simulink model "QPSK_Transmit_v5_w_FIFO_w_errors"  (R2012b)
settings: Solver=FixedStepDiscrete  StartTime=0.0  StopTime=1500  FixedStep=1  RelTol=1e-3
libraries: simulink x14, dspbuff3 x1, commutil2 x1
settings Model: Creator=Carl  LastModifiedBy=Carl
settings DataIOCC: SignalLogging=off
settings OptimizationCC: BlockReduction=off  ConditionallyExecuteInputs=off  InlineParams=on
settings DebuggingCC: AlgebraicLoopMsg=error
settings HardwareCC: ProdHWDeviceType=ASIC/FPGA->ASIC/FPGA  ProdEqTarget=off

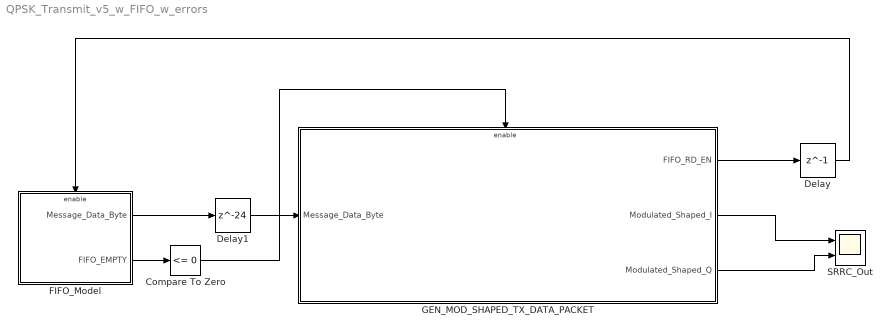
== system QPSK_Transmit_v5_w_FIFO_w_errors ==
  Compare To Zero : simulink/Logic and Bit Operations/Compare To Zero  relop=<=  OutDataTypeStr=boolean
  Delay : Delay  DelayLength=1  InitialCondition=0
  Delay1 : Delay  DelayLength=24  InitialCondition=0
  FIFO_Model : Subsystem
  GEN_MOD_SHAPED_TX_DATA_PACKET : Subsystem
  SRRC_Out : Scope  NumInputPorts=2
      settings: YMin=-5~-5  YMax=5~5  SaveName=ScopeData7
  wires:
  GEN_MOD_SHAPED_TX_DATA_PACKET/2(Modulated_Shaped_I) -> SRRC_Out/1
  GEN_MOD_SHAPED_TX_DATA_PACKET/3(Modulated_Shaped_Q) -> SRRC_Out/2
  GEN_MOD_SHAPED_TX_DATA_PACKET/1(FIFO_RD_EN) -> Delay/1
  Delay/1 -> FIFO_Model/Enable
  FIFO_Model/2(FIFO_EMPTY) -> Compare To Zero/1
  Compare To Zero/1 -> GEN_MOD_SHAPED_TX_DATA_PACKET/Enable
  FIFO_Model/1(Message_Data_Byte) -> Delay1/1
  Delay1/1 -> GEN_MOD_SHAPED_TX_DATA_PACKET/1(Message_Data_Byte)

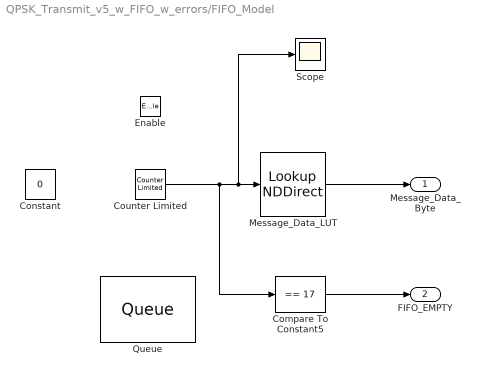
== system QPSK_Transmit_v5_w_FIFO_w_errors/FIFO_Model ==
  Enable : EnablePort
  Compare To Constant5 : simulink/Logic and Bit Operations/Compare To Constant  relop===  const=17  OutDataTypeStr=boolean  ZeroCross=off
  Constant : Constant  Value=0
  Counter Limited : simulink/Sources/Counter Limited  uplimit=17  tsamp=-1
  Message_Data_LUT : LookupNDDirect  NumberOfTableDimensions=1  Table="[12        0        0        1        104        101        108        108        111        32        119        111        114        108        100        33        198        228]"  DiagnosticForOutOfRangeInput=Error  TableDataTypeStr=uint8
  Queue : dspbuff3/Queue  depth=8  trigger=Rising edge  overflow=Dynamic reallocation  pes=Warning  eso=off  fso=off  nso=off  clr=off  clrOutport=off  adf=on
  Scope : Scope
  Message_Data_Byte : Outport
  FIFO_EMPTY : Outport  Port=2
  wires:
  Message_Data_LUT/1 -> Message_Data_Byte/1
  Counter Limited/1 -> Compare To Constant5/1, Scope/1, Message_Data_LUT/1
  Compare To Constant5/1 -> FIFO_EMPTY/1

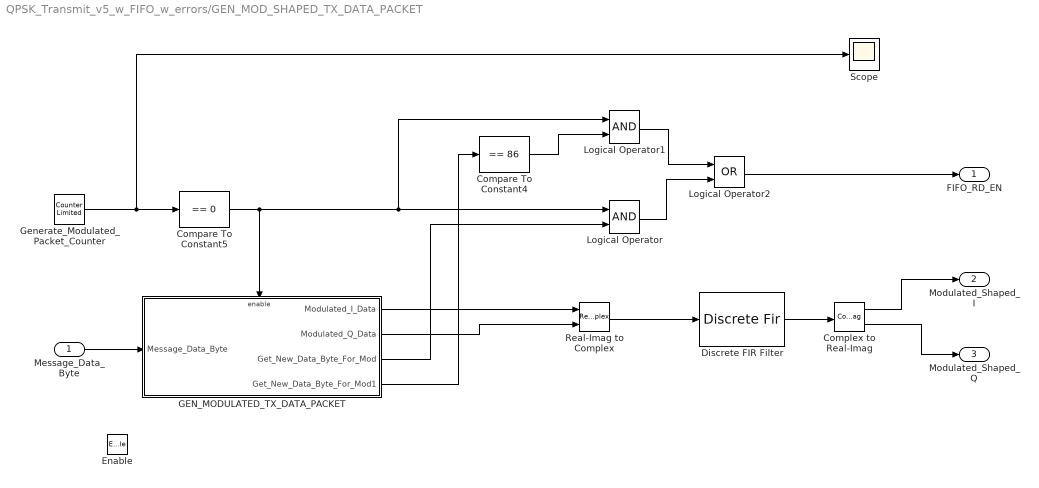
== system QPSK_Transmit_v5_w_FIFO_w_errors/GEN_MOD_SHAPED_TX_DATA_PACKET ==
  Message_Data_Byte : Inport
  Enable : EnablePort
  Compare To Constant4 : simulink/Logic and Bit Operations/Compare To Constant  relop===  const=86  OutDataTypeStr=boolean  ZeroCross=off
  Compare To Constant5 : simulink/Logic and Bit Operations/Compare To Constant  relop===  const=0  OutDataTypeStr=boolean  ZeroCross=off
  Complex to Real-Imag : ComplexToRealImag
  Discrete FIR Filter : DiscreteFir  Coefficients=|
      | [
      | 0.006690562067
      | -0.005768593810
      | -0.011827354519
      | 0.020586915021
      | 0.016726405168
      | -0.053692342207
      | -0.020253031546
      | 0.196043589067
      | 0.336822413190
      | 0.196043589067
      | -0.020253031546
      | -0.053692342207
      | 0.016726405168
      | 0.020586915021
      | -0.011827354519
      | -0.005768593810
      | 0.006690562067
      | ]
  GEN_MODULATED_TX_DATA_PACKET : Subsystem
  Generate_Modulated_Packet_Counter : simulink/Sources/Counter Limited  uplimit=7  tsamp=-1
  Logical Operator : Logic  AllPortsSameDT=off  OutDataTypeStr=boolean
  Logical Operator1 : Logic  AllPortsSameDT=off  OutDataTypeStr=boolean
  Logical Operator2 : Logic  Operator=OR  AllPortsSameDT=off  OutDataTypeStr=boolean
  Real-Imag to Complex : RealImagToComplex
  Scope : Scope
      settings: SaveName=ScopeData10
  FIFO_RD_EN : Outport
  Modulated_Shaped_I : Outport  Port=2
  Modulated_Shaped_Q : Outport  Port=3
  wires:
  Real-Imag to Complex/1 -> Discrete FIR Filter/1
  Discrete FIR Filter/1 -> Complex to Real-Imag/1
  Complex to Real-Imag/1 -> Modulated_Shaped_I/1
  Complex to Real-Imag/2 -> Modulated_Shaped_Q/1
  GEN_MODULATED_TX_DATA_PACKET/1(Modulated_I_Data) -> Real-Imag to Complex/1
  GEN_MODULATED_TX_DATA_PACKET/2(Modulated_Q_Data) -> Real-Imag to Complex/2
  Generate_Modulated_Packet_Counter/1 -> Scope/1, Compare To Constant5/1
  Message_Data_Byte/1 -> GEN_MODULATED_TX_DATA_PACKET/1(Message_Data_Byte)
  GEN_MODULATED_TX_DATA_PACKET/3(Get_New_Data_Byte_For_Mod) -> Logical Operator/2
  Compare To Constant5/1 -> GEN_MODULATED_TX_DATA_PACKET/Enable, Logical Operator1/1, Logical Operator/1
  Compare To Constant4/1 -> Logical Operator1/2
  GEN_MODULATED_TX_DATA_PACKET/4(Get_New_Data_Byte_For_Mod1) -> Compare To Constant4/1
  Logical Operator/1 -> Logical Operator2/2
  Logical Operator1/1 -> Logical Operator2/1
  Logical Operator2/1 -> FIFO_RD_EN/1

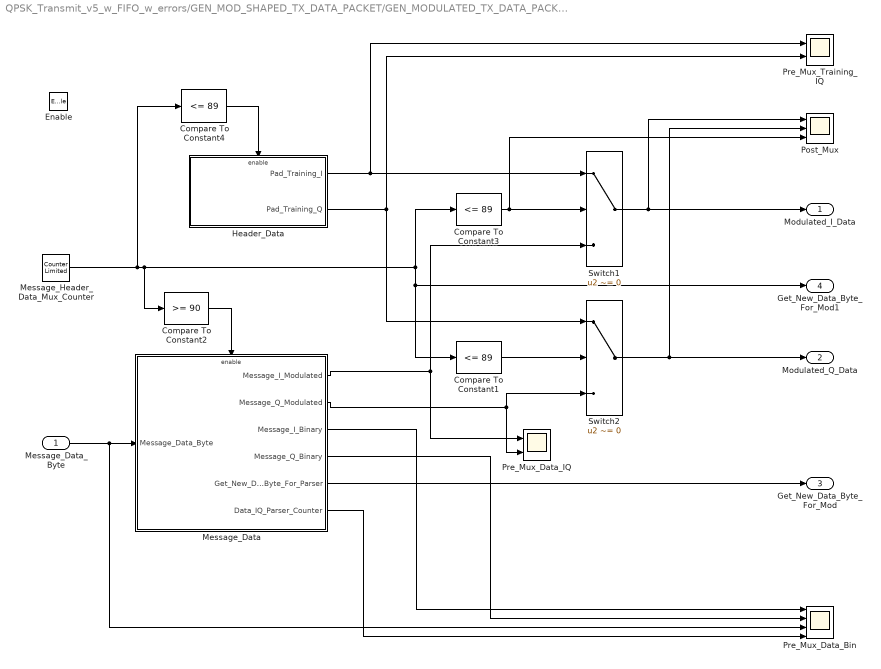
== system QPSK_Transmit_v5_w_FIFO_w_errors/GEN_MOD_SHAPED_TX_DATA_PACKET/GEN_MODULATED_TX_DATA_PACKET ==
  Message_Data_Byte : Inport
  Enable : EnablePort
  Compare To Constant1 : simulink/Logic and Bit Operations/Compare To Constant  relop=<=  const=89  OutDataTypeStr=boolean  ZeroCross=off
  Compare To Constant2 : simulink/Logic and Bit Operations/Compare To Constant  relop=>=  const=90  OutDataTypeStr=boolean  ZeroCross=off
  Compare To Constant3 : simulink/Logic and Bit Operations/Compare To Constant  relop=<=  const=89  OutDataTypeStr=boolean  ZeroCross=off
  Compare To Constant4 : simulink/Logic and Bit Operations/Compare To Constant  relop=<=  const=89  OutDataTypeStr=boolean  ZeroCross=off
  Header_Data : Subsystem
  Message_Data : Subsystem
  Message_Header_Data_Mux_Counter : simulink/Sources/Counter Limited  uplimit=1023  tsamp=-1
  Post_Mux : Scope  NumInputPorts=3
      settings: YMin=-5~-5~-5  YMax=5~5~5  SaveName=ScopeData2
  Pre_Mux_Data_Bin : Scope  NumInputPorts=4
      settings: TimeRange=1500  YMin=-0.2~-0.2~-10~-5  YMax=1.2~1.2~265~5  SaveName=ScopeData6
  Pre_Mux_Data_IQ : Scope  NumInputPorts=2
      settings: YMin=-5~-5  YMax=5~5  SaveName=ScopeData5
  Pre_Mux_Training_IQ : Scope  NumInputPorts=2
      settings: YMin=-5~-5  YMax=5~5  SaveName=ScopeData4
  Switch1 : Switch  Criteria=u2 ~= 0  OutDataTypeStr=int8
  Switch2 : Switch  Criteria=u2 ~= 0  OutDataTypeStr=int8
  Modulated_I_Data : Outport
  Modulated_Q_Data : Outport  Port=2
  Get_New_Data_Byte_For_Mod : Outport  Port=3
  Get_New_Data_Byte_For_Mod1 : Outport  Port=4
  wires:
  Message_Header_Data_Mux_Counter/1 -> Compare To Constant4/1, Compare To Constant3/1, Get_New_Data_Byte_For_Mod1/1, Compare To Constant1/1, Compare To Constant2/1
  Switch1/1 -> Modulated_I_Data/1, Post_Mux/1
  Header_Data/1(Pad_Training_I) -> Switch1/1, Pre_Mux_Training_IQ/1
  Compare To Constant1/1 -> Switch2/2
  Switch2/1 -> Post_Mux/2, Modulated_Q_Data/1
  Header_Data/2(Pad_Training_Q) -> Switch2/1, Pre_Mux_Training_IQ/2
  Message_Data/2(Message_Q_Modulated) -> Pre_Mux_Data_IQ/2, Switch2/3
  Message_Data/1(Message_I_Modulated) -> Pre_Mux_Data_IQ/1, Switch1/3
  Message_Data/3(Message_I_Binary) -> Pre_Mux_Data_Bin/1
  Message_Data/4(Message_Q_Binary) -> Pre_Mux_Data_Bin/2
  Compare To Constant2/1 -> Message_Data/Enable
  Compare To Constant4/1 -> Header_Data/Enable
  Message_Data_Byte/1 -> Pre_Mux_Data_Bin/3, Message_Data/1(Message_Data_Byte)
  Compare To Constant3/1 -> Post_Mux/3, Switch1/2
  Message_Data/5(Get_New_Data_Byte_For_Parser) -> Get_New_Data_Byte_For_Mod/1
  Message_Data/6(Data_IQ_Parser_Counter) -> Pre_Mux_Data_Bin/4

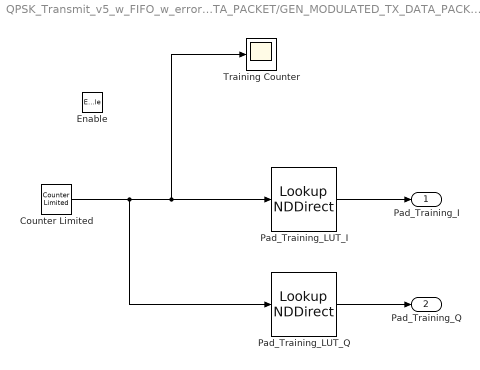
== system QPSK_Transmit_v5_w_FIFO_w_errors/GEN_MOD_SHAPED_TX_DATA_PACKET/GEN_MODULATED_TX_DATA_PACKET/Header_Data ==
  Enable : EnablePort
  Counter Limited : simulink/Sources/Counter Limited  uplimit=89  tsamp=-1
  Pad_Training_LUT_I : LookupNDDirect  NumberOfTableDimensions=1  Table=[1,-1,1,-1,1,-1,1,-1,1,-1,1,-1,1,-1,1,-1,1,-1,1,-1,1,-1,1,-1,1,1,1,-1,-1,1,1,-1,-1,1,-1,-1,-1,-1,1,-1,1,1,-1,-1,1,1,1,-1,1,1,1,-1,1,-1,1,1,1,-1,1,1,1,1,-1,1,1,-1,-1,-1,-1,1,1,1,-1,-1,-1,1,1,1,1,-1,1,1,1,1,1,-1,-1,-1,1,1]  DiagnosticForOutOfRangeInput=Error  TableDataTypeStr=int8
  Pad_Training_LUT_Q : LookupNDDirect  NumberOfTableDimensions=1  Table=[1,-1,1,-1,1,-1,1,-1,1,-1,1,-1,1,-1,1,-1,1,-1,1,-1,1,-1,1,-1,1,1,-1,1,1,1,-1,-1,-1,-1,1,1,-1,1,1,-1,-1,-1,1,-1,-1,1,1,1,-1,-1,1,1,1,-1,-1,-1,-1,-1,-1,1,1,-1,1,-1,1,1,-1,-1,1,-1,-1,1,1,-1,-1,-1,-1,-1,1,1,1,1,-1,-1,-1,-1,1,-1,1,-1]  DiagnosticForOutOfRangeInput=Error  TableDataTypeStr=int8
  Training Counter : Scope
      settings: SaveName=ScopeData3
  Pad_Training_I : Outport
  Pad_Training_Q : Outport  Port=2
  wires:
  Pad_Training_LUT_I/1 -> Pad_Training_I/1
  Counter Limited/1 -> Training Counter/1, Pad_Training_LUT_I/1, Pad_Training_LUT_Q/1
  Pad_Training_LUT_Q/1 -> Pad_Training_Q/1

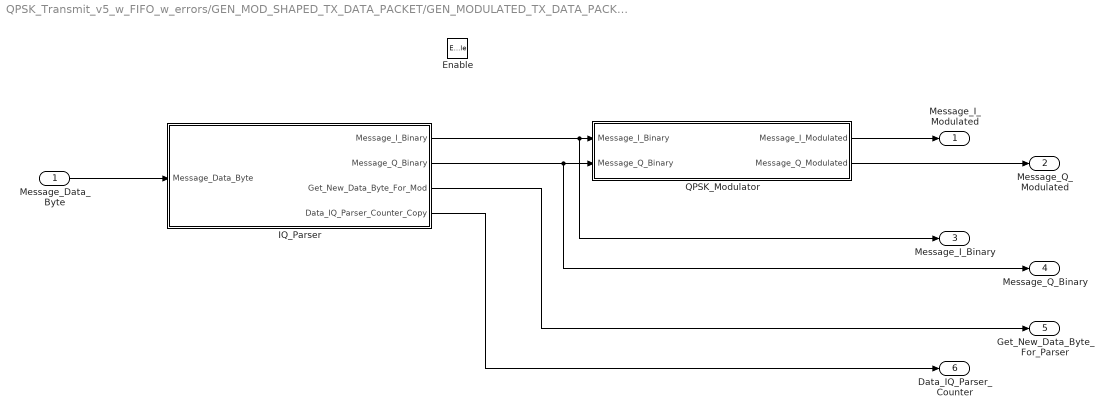
== system QPSK_Transmit_v5_w_FIFO_w_errors/GEN_MOD_SHAPED_TX_DATA_PACKET/GEN_MODULATED_TX_DATA_PACKET/Message_Data ==
  Message_Data_Byte : Inport
  Enable : EnablePort
  IQ_Parser : Subsystem
  QPSK_Modulator : Subsystem
  Message_I_Modulated : Outport
  Message_Q_Modulated : Outport  Port=2
  Message_I_Binary : Outport  Port=3
  Message_Q_Binary : Outport  Port=4
  Get_New_Data_Byte_For_Parser : Outport  Port=5
  Data_IQ_Parser_Counter : Outport  Port=6
  wires:
  IQ_Parser/1(Message_I_Binary) -> Message_I_Binary/1, QPSK_Modulator/1(Message_I_Binary)
  IQ_Parser/2(Message_Q_Binary) -> Message_Q_Binary/1, QPSK_Modulator/2(Message_Q_Binary)
  QPSK_Modulator/1(Message_I_Modulated) -> Message_I_Modulated/1
  QPSK_Modulator/2(Message_Q_Modulated) -> Message_Q_Modulated/1
  Message_Data_Byte/1 -> IQ_Parser/1(Message_Data_Byte)
  IQ_Parser/3(Get_New_Data_Byte_For_Mod) -> Get_New_Data_Byte_For_Parser/1
  IQ_Parser/4(Data_IQ_Parser_Counter_Copy) -> Data_IQ_Parser_Counter/1

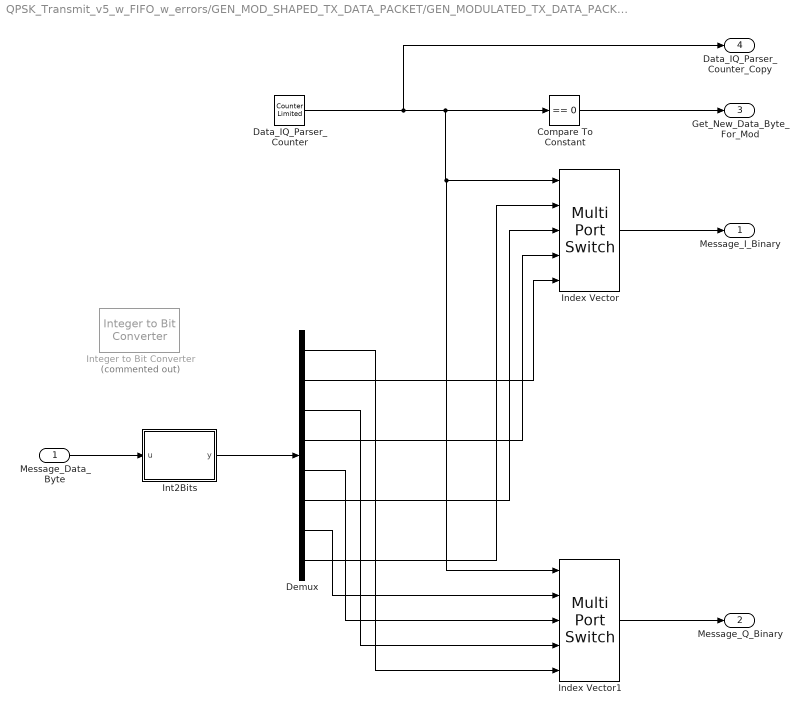
== system QPSK_Transmit_v5_w_FIFO_w_errors/GEN_MOD_SHAPED_TX_DATA_PACKET/GEN_MODULATED_TX_DATA_PACKET/Message_Data/IQ_Parser ==
  Message_Data_Byte : Inport
  Compare To Constant : simulink/Logic and Bit Operations/Compare To Constant  relop===  const=0  OutDataTypeStr=boolean
  Data_IQ_Parser_Counter : simulink/Sources/Counter Limited  uplimit=3  tsamp=-1
  Demux : Demux  Outputs=8
  Index Vector : MultiPortSwitch  DataPortOrder=Zero-based contiguous  Inputs=4  zeroidx=on
  Index Vector1 : MultiPortSwitch  DataPortOrder=Zero-based contiguous  Inputs=4  zeroidx=on
  Int2Bits : MATLAB Function  TreatAsAtomicUnit=on
  Integer to Bit Converter : commutil2/Integer to Bit Converter  Commented=on  nbits=8  signedInputValues=Unsigned  bitOrder=MSB first  outDtype=Inherit via internal rule
  Message_I_Binary : Outport
  Message_Q_Binary : Outport  Port=2
  Get_New_Data_Byte_For_Mod : Outport  Port=3
  Data_IQ_Parser_Counter_Copy : Outport  Port=4
  wires:
  Index Vector1/1 -> Message_Q_Binary/1
  Data_IQ_Parser_Counter/1 -> Data_IQ_Parser_Counter_Copy/1, Compare To Constant/1, Index Vector/1, Index Vector1/1
  Index Vector/1 -> Message_I_Binary/1
  Demux/8 -> Index Vector/2
  Demux/7 -> Index Vector1/2
  Demux/6 -> Index Vector/3
  Demux/5 -> Index Vector1/3
  Demux/4 -> Index Vector/4
  Demux/3 -> Index Vector1/4
  Demux/2 -> Index Vector/5
  Demux/1 -> Index Vector1/5
  Message_Data_Byte/1 -> Int2Bits/1(u)
  Int2Bits/1(y) -> Demux/1
  Compare To Constant/1 -> Get_New_Data_Byte_For_Mod/1

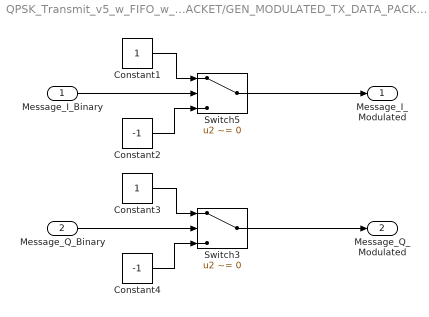
== system QPSK_Transmit_v5_w_FIFO_w_errors/GEN_MOD_SHAPED_TX_DATA_PACKET/GEN_MODULATED_TX_DATA_PACKET/Message_Data/QPSK_Modulator ==
  Message_I_Binary : Inport
  Message_Q_Binary : Inport  Port=2
  Constant1 : Constant  OutDataTypeStr=int8
  Constant2 : Constant  Value=-1  OutDataTypeStr=int8
  Constant3 : Constant  OutDataTypeStr=int8
  Constant4 : Constant  Value=-1  OutDataTypeStr=int8
  Switch3 : Switch  Criteria=u2 ~= 0  RndMeth=Round
  Switch5 : Switch  Criteria=u2 ~= 0  RndMeth=Round
  Message_I_Modulated : Outport
  Message_Q_Modulated : Outport  Port=2
  wires:
  Switch3/1 -> Message_Q_Modulated/1
  Constant4/1 -> Switch3/3
  Constant2/1 -> Switch5/3
  Constant1/1 -> Switch5/1
  Message_Q_Binary/1 -> Switch3/2
  Constant3/1 -> Switch3/1
  Switch5/1 -> Message_I_Modulated/1
  Message_I_Binary/1 -> Switch5/2

== matlab function QPSK_Transmit_v5_w_FIFO_w_errors/GEN_MOD_SHAPED_TX_DATA_PACKET/GEN_MODULATED_TX_DATA_PACKET/Message_Data/IQ_Parser/Int2Bits ==
  data: u input; y output
function y = fcn(u)
% Converts Integer(8bits) to a 1-D array Bits

y = bitget(u, [8:-1:1])';
